simulink model "mySunroof"  (R2020b)
settings: Solver=VariableStepAuto  StartTime=0.0  StopTime=inf  RelTol=1e-3
settings Model: Creator=kumar  LastModifiedBy=99003745

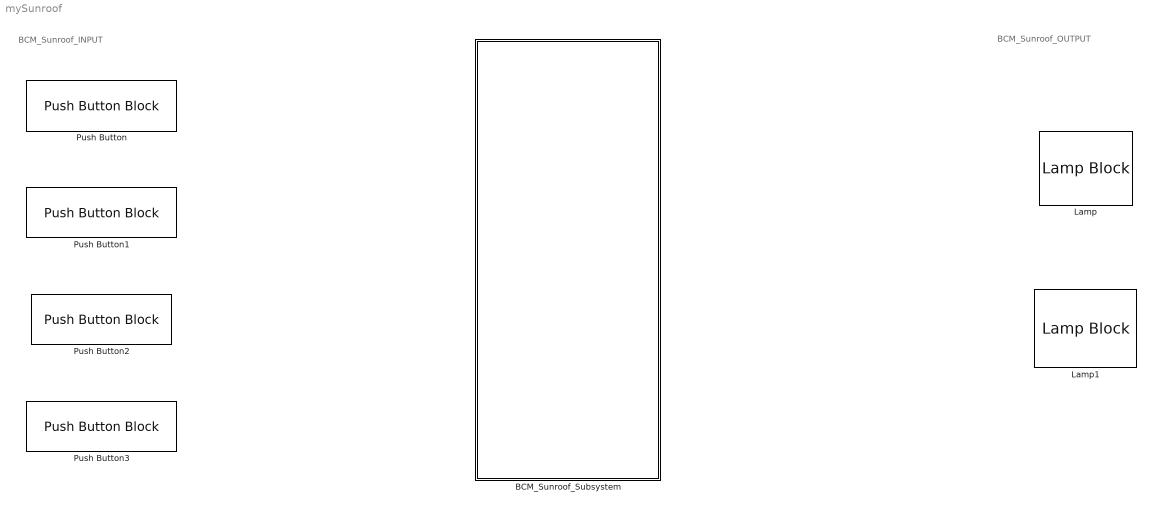
== system mySunroof ==
  note: BCM_Sunroof_OUTPUT
  note: BCM_Sunroof_INPUT
  BCM_Sunroof_Subsystem : Subsystem
  Lamp : LampBlock  LabelPosition=Bottom
  Lamp1 : LampBlock  LabelPosition=Bottom
  Push Button : PushButtonBlock  ButtonText=BCM_Sunroof_SlideON
  Push Button1 : PushButtonBlock  ButtonText=BCM_Sunroof_Stop
  Push Button2 : PushButtonBlock  ButtonText=BCM_Sunroof_SlideOFF
  Push Button3 : PushButtonBlock  ButtonText=BCM_Sunroof_Obstacle

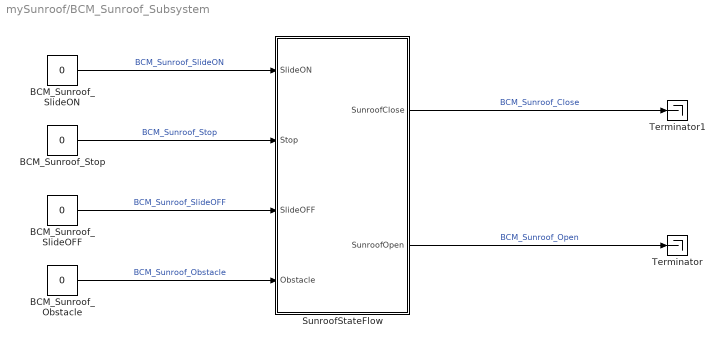
== system mySunroof/BCM_Sunroof_Subsystem ==
  BCM_Sunroof_Obstacle : Constant  Value=0
  BCM_Sunroof_SlideOFF : Constant  Value=0
  BCM_Sunroof_SlideON : Constant  Value=0
  BCM_Sunroof_Stop : Constant  Value=0
  SunroofStateFlow : Stateflow chart  TreatAsAtomicUnit=on
  Terminator : Terminator
  Terminator1 : Terminator
  wires:
  BCM_Sunroof_SlideON/1 -> SunroofStateFlow/1(SlideON)  "BCM_Sunroof_SlideON"
  BCM_Sunroof_SlideOFF/1 -> SunroofStateFlow/3(SlideOFF)  "BCM_Sunroof_SlideOFF"
  BCM_Sunroof_Stop/1 -> SunroofStateFlow/2(Stop)  "BCM_Sunroof_Stop"
  SunroofStateFlow/1(SunroofClose) -> Terminator1/1  "BCM_Sunroof_Close"
  BCM_Sunroof_Obstacle/1 -> SunroofStateFlow/4(Obstacle)  "BCM_Sunroof_Obstacle"
  SunroofStateFlow/2(SunroofOpen) -> Terminator/1  "BCM_Sunroof_Open"

== stateflow chart mySunroof/BCM_Sunroof_Subsystem/SunroofStateFlow ==
  state safe
    state SunroofState
      entry:
      SunroofOpen=0;
      SunroofClose=0;
      state Switch
        entry:
        SunroofOpen=0;
        SunroofClose=0;
      state Sunroofopen
        entry: SunroofOpen=1;
        exit: SunroofOpen=0;
        state iniSunroofOpen
      state SunroofClose
        entry: SunroofClose=1;
        exit: SunroofClose=0;
        state iniSunroofClose
      Switch -> iniSunroofClose [order 2] : [SlideOFF==1]
      Switch -> iniSunroofOpen [order 1] : [SlideON==1]
      Sunroofopen -> Switch [order 1] : [Stop]
      SunroofClose -> Switch [order 1] : [Stop]
      SunroofClose -> Sunroofopen [order 2] : [SlideON==1]
      Sunroofopen -> SunroofClose [order 2] : [SlideOFF==1]
    (default) -> Switch
  state EmergencyOpen
    entry:
    SunroofOpen=1;
    SunroofClose=0;
  (default) -> safe [order 1]
  (default) -> SunroofState [order 2]
  EmergencyOpen -> Switch : [Stop||SlideOFF]
  safe -> EmergencyOpen : [Obstacle==1]
  data: SlideON input; Stop input; SlideOFF input; Obstacle input; SunroofClose output; SunroofOpen output
